simulink model "pipeline_sar_adc_v2"  (R2026a)
settings: Solver=FixedStepDiscrete  FixedStep=1e-9
values from neighbouring files (symbols this model uses):
  bit_1st = 6    [script_MonteCarlo.m]    (also in script_MonteCarlo_v2.m; script_spectrum.m; script_spectrum_v2.m)
  bit_2nd = 9    [script_MonteCarlo.m]    (also in script_MonteCarlo_v2.m; script_spectrum.m; script_spectrum_v2.m)
  CDAC_skew = 10e-9    (= 1e-08)    [script_MonteCarlo_v2.m]    (also in script_spectrum_v2.m = 1e-09)
  CMPno_1st = 0    [script_MonteCarlo.m]    (also in script_MonteCarlo_v2.m; script_spectrum.m; script_spectrum_v2.m)
  CMPno_2nd = 0    [script_MonteCarlo.m]    (also in script_MonteCarlo_v2.m; script_spectrum.m; script_spectrum_v2.m)
  CMPoff_1st = 0    [script_MonteCarlo.m]    (also in script_MonteCarlo_v2.m; script_spectrum.m; script_spectrum_v2.m)
  CMPoff_2nd = 0    [script_MonteCarlo.m]    (also in script_MonteCarlo_v2.m; script_spectrum.m; script_spectrum_v2.m)
  DAC_1st = DAC_1st_scaled(1 : (bit_1st + 1)) / (2^bit_1st)    [script_MonteCarlo.m]    (also in script_MonteCarlo_v2.m = DAC_1st_scaled(1 : bit_1st) / (2^(bit_1st-1)); script_spectrum.m; script_spectrum_v2.m = DAC_1st_scaled(1 : bit_1st) / (2^(bit_1st-1)))
  DAC_1st_v2 = DAC_big_scaled(1 : (bit_1st + 1)) / (2^bit_1st)    [script_MonteCarlo_v2.m]    (also in script_spectrum_v2.m)
  DAC_2nd = 0    [script_MonteCarlo.m]    (also in script_MonteCarlo_v2.m; script_spectrum.m; script_spectrum_v2.m)
  fin = (M / N) * fs    (= 488281.25)    [script_MonteCarlo.m]    (also in script_MonteCarlo_v2.m; script_spectrum.m; script_spectrum_v2.m = 292968.75)
  fs = 100e6    (= 100000000)    [script_MonteCarlo.m]    (also in script_MonteCarlo_v2.m; script_spectrum.m; script_spectrum_v2.m)
  mean_kTC = 0    [script_MonteCarlo.m]    (also in script_MonteCarlo_v2.m; script_spectrum.m; script_spectrum_v2.m)
  seed_kTC_1st = randi(1e6)    [script_MonteCarlo.m]    (also in script_MonteCarlo_v2.m; script_spectrum.m; script_spectrum_v2.m = randi(2^31))
  seed_kTC_2nd = randi(1e6)    [script_MonteCarlo.m]    (also in script_MonteCarlo_v2.m; script_spectrum.m; script_spectrum_v2.m = randi(2^31))
  seed_kTC_big = randi(1e6)    [script_MonteCarlo_v2.m]    (also in script_spectrum_v2.m = randi(2^31))
  var_kTC_1st = kTC_en_1st * sigma_kTC_1st^2    [script_MonteCarlo.m]    (also in script_MonteCarlo_v2.m; script_spectrum.m; script_spectrum_v2.m)
  var_kTC_2nd = kTC_en_2nd * sigma_kTC_2nd^2    [script_MonteCarlo.m]    (also in script_MonteCarlo_v2.m; script_spectrum.m; script_spectrum_v2.m)
  var_kTC_big = kTC_en_big * sigma_kTC_big^2    [script_MonteCarlo_v2.m]    (also in script_spectrum_v2.m)
  Vin = 0.95    [script_MonteCarlo.m]    (also in script_MonteCarlo_v2.m; script_parametric_analysis.m = Vin_array(idx); script_spectrum.m; script_spectrum_v2.m)
settings Model: Creator=오지훈  LastModifiedBy=오지훈

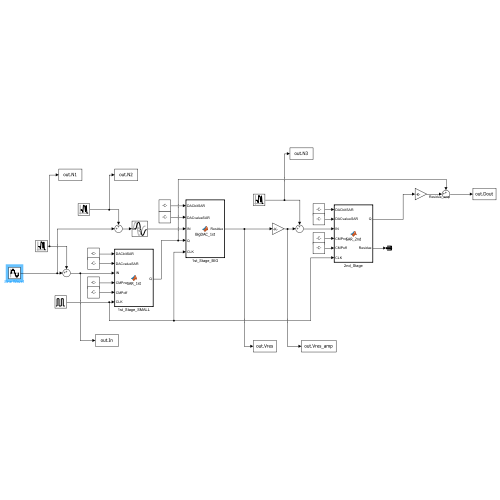
[thumbnail: Simulink's stored preview of the top-level diagram]
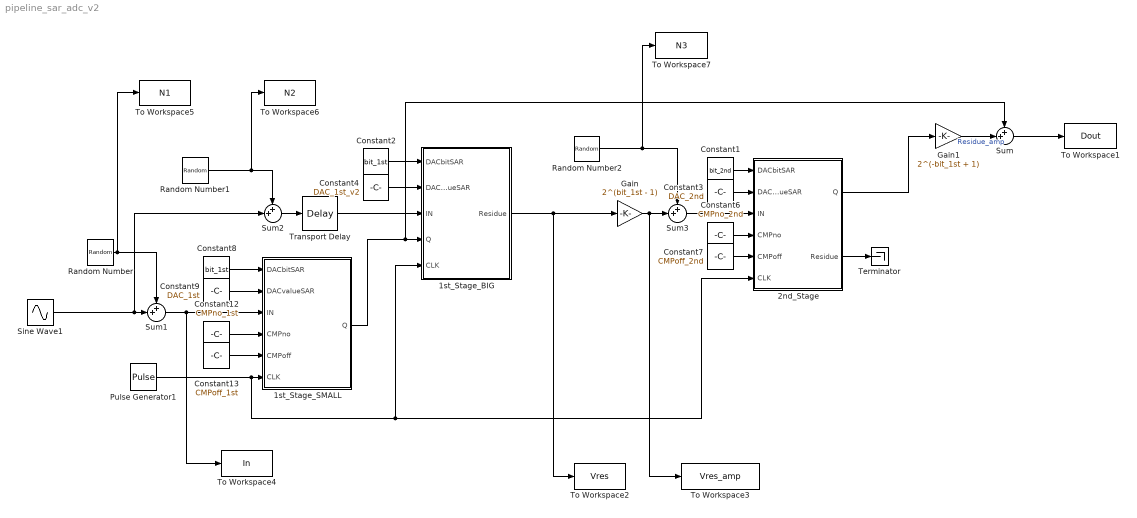
== system pipeline_sar_adc_v2 ==
  1st_Stage_BIG : MATLAB Function  TreatAsAtomicUnit=on
  1st_Stage_SMALL : MATLAB Function  TreatAsAtomicUnit=on
  2nd_Stage : MATLAB Function  TreatAsAtomicUnit=on
  Constant1 : Constant  Value=bit_2nd
  Constant12 : Constant  Value=CMPno_1st
  Constant13 : Constant  Value=CMPoff_1st
  Constant2 : Constant  Value=bit_1st
  Constant3 : Constant  Value=DAC_2nd
  Constant4 : Constant  Value=DAC_1st_v2
  Constant6 : Constant  Value=CMPno_2nd
  Constant7 : Constant  Value=CMPoff_2nd
  Constant8 : Constant  Value=bit_1st
  Constant9 : Constant  Value=DAC_1st
  Gain : Gain  Gain=2^(bit_1st - 1)
  Gain1 : Gain  Gain=2^(-bit_1st + 1)
  Pulse Generator1 : DiscretePulseGenerator  PulseType=Time based  Period=1/fs  PulseWidth=50
  Random Number : RandomNumber  Mean=mean_kTC  Variance=var_kTC_1st  Seed=seed_kTC_1st  SampleTime=1/fs
  Random Number1 : RandomNumber  Mean=mean_kTC  Variance=var_kTC_big  Seed=seed_kTC_big  SampleTime=1/fs
  Random Number2 : RandomNumber  Mean=mean_kTC  Variance=var_kTC_2nd  Seed=seed_kTC_2nd  SampleTime=1/fs
  Sine Wave1 : Sin  Amplitude=Vin  Frequency=2*pi*fin  SampleTime=CDAC_skew
  Sum{,1..3} (4 alike) : Sum  Inputs=++|
  Terminator : Terminator
  To Workspace1 : ToWorkspace  VariableName=Dout  SaveFormat=Timeseries  SampleTime=1/fs
  To Workspace2 : ToWorkspace  VariableName=Vres  SaveFormat=Timeseries  SampleTime=1/fs
  To Workspace3 : ToWorkspace  VariableName=Vres_amp  SaveFormat=Timeseries  SampleTime=1/fs
  To Workspace4 : ToWorkspace  VariableName=In  SaveFormat=Timeseries  SampleTime=1/fs
  To Workspace5 : ToWorkspace  VariableName=N1  SaveFormat=Timeseries  SampleTime=1/fs
  To Workspace6 : ToWorkspace  VariableName=N2  SaveFormat=Timeseries  SampleTime=1/fs
  To Workspace7 : ToWorkspace  VariableName=N3  SaveFormat=Timeseries  SampleTime=1/fs
  Transport Delay : TransportDelay  DelayTime=CDAC_skew
  wires:
  Sum1/1 -> To Workspace4/1, 1st_Stage_SMALL/3(IN)
  2nd_Stage/2(Residue) -> Terminator/1
  Constant3/1 -> 2nd_Stage/2(DACvalueSAR)
  Constant4/1 -> 1st_Stage_BIG/2(DACvalueSAR)
  Constant2/1 -> 1st_Stage_BIG/1(DACbitSAR)
  1st_Stage_BIG/1(Residue) -> Gain/1, To Workspace2/1
  Constant1/1 -> 2nd_Stage/1(DACbitSAR)
  Constant7/1 -> 2nd_Stage/5(CMPoff)
  Constant13/1 -> 1st_Stage_SMALL/5(CMPoff)
  Constant6/1 -> 2nd_Stage/4(CMPno)
  Sum/1 -> To Workspace1/1
  Constant12/1 -> 1st_Stage_SMALL/4(CMPno)
  Constant9/1 -> 1st_Stage_SMALL/2(DACvalueSAR)
  Gain/1 -> To Workspace3/1, Sum3/2
  Gain1/1 -> Sum/2  "Residue_amp"
  Constant8/1 -> 1st_Stage_SMALL/1(DACbitSAR)
  2nd_Stage/1(Q) -> Gain1/1
  Pulse Generator1/1 -> 2nd_Stage/6(CLK), 1st_Stage_BIG/5(CLK), 1st_Stage_SMALL/6(CLK)
  1st_Stage_SMALL/1(Q) -> 1st_Stage_BIG/4(Q), Sum/1
  Sine Wave1/1 -> Sum2/2, Sum1/2
  Random Number/1 -> To Workspace5/1, Sum1/1
  Sum2/1 -> Transport Delay/1
  Random Number1/1 -> To Workspace6/1, Sum2/1
  Sum3/1 -> 2nd_Stage/3(IN)
  Random Number2/1 -> To Workspace7/1, Sum3/1
  Transport Delay/1 -> 1st_Stage_BIG/3(IN)

== matlab function pipeline_sar_adc_v2/1st_Stage_SMALL ==
  data: DACbitSAR input; Q output; DACvalueSAR input; IN input; CMPno input; CMPoff input; CLK input
function Q = SAR_1st(DACbitSAR, DACvalueSAR, IN, CMPno, CMPoff, CLK)
persistent last_CLK Q_hold
if isempty(last_CLK)
    last_CLK = 0;
    Q_hold = 0;
end
if (last_CLK == 0) && (CLK == 1)
    current_residue = IN;
    Q_partial_sum = 0;
    len_DAC = length(DACvalueSAR);
    
    % --- SAR 5번 판정 (residue 5번 갱신) ---
    for i = 1:DACbitSAR-1
        CMP_threshold = CMPno * randn(1) + CMPoff;
        current_idx = len_DAC - i + 1;
        current_dac = DACvalueSAR(current_idx);
        bit_weight = 2^(-(i-1));
        if current_residue >= CMP_threshold
            current_residue = current_residue - current_dac;
            Q_partial_sum = Q_partial_sum + 1 * bit_weight;
        else
            current_residue = current_residue + current_dac;
        end
    end
    
    % --- Residue 확정 후 마지막 판정 (Q에만 반영, residue 갱신 없음) ---
    CMP_threshold = CMPno * randn(1) + CMPoff;
    bit_weight = 2^(-(DACbitSAR-1));   % 마지막 bit weight = 2^-5
    if current_residue >= CMP_threshold
        Q_partial_sum = Q_partial_sum + 1 * bit_weight;
    end
    
    Q_hold = Q_partial_sum - 1;
end
Q = Q_hold;
last_CLK = CLK;
end

== matlab function pipeline_sar_adc_v2/1st_Stage_BIG ==
  data: DACbitSAR input; DACvalueSAR input; IN input; Q input; Residue output; CLK input
function Residue = BigDAC_1st(DACbitSAR, DACvalueSAR, IN, Q, CLK)
% Big DAC (1st stage) — 판정 없음. Small DAC의 코드(Q)를 받아 residue만 생성.
% 에러: 커패시터 미스매치(DACvalueSAR에 반영).
% 비교기 offset/noise 없음 (이 블록에는 비교기가 없음).
persistent last_CLK Residue_hold
if isempty(last_CLK)
    last_CLK = 0;
    Residue_hold = 0;
end

if (last_CLK == 0) && (CLK == 1)
    current_residue = IN;
    len_DAC = length(DACvalueSAR);

    % ---- Q로부터 Small DAC의 비트 결정을 복원 (재비교 안 함) ----
    Q_partial_sum = Q + 1;              % small의 -1 스케일링 역산
    remaining = Q_partial_sum;

    for i = 1:DACbitSAR
        bit_weight = 2^(-(i-1));
        current_idx = len_DAC - i + 1;
        current_dac = DACvalueSAR(current_idx);   % 미스매치 포함 실제 값

        % small이 이 비트를 1로 정했는지 복원
        if remaining >= bit_weight
            bit = 1;
            remaining = remaining - bit_weight;
        else
            bit = 0;
        end

        % small의 결정 그대로 따라 residue 갱신
        if bit == 1
            current_residue = current_residue - current_dac;
        else
            current_residue = current_residue + current_dac;
        end
    end

    Residue_hold = current_residue;
end

Residue = Residue_hold;
last_CLK = CLK;
end

== matlab function pipeline_sar_adc_v2/2nd_Stage ==
  data: DACbitSAR input; Q output; DACvalueSAR input; IN input; CMPno input; CMPoff input; Residue output; CLK input
function [Q, Residue] = SAR_2nd(DACbitSAR, DACvalueSAR, IN, CMPno, CMPoff, CLK)
persistent last_CLK Q_hold Residue_hold

if isempty(last_CLK)
    last_CLK = 0;
    Q_hold = 0;
    Residue_hold = 0;
end

if (last_CLK == 0) && (CLK == 1)
    
    current_residue = IN; 
    Q_partial_sum = 0;    % ★ Partial sum을 누적할 변수 초기화
    len_DAC = length(DACvalueSAR); 
    
    for i = 1:DACbitSAR
        CMP_threshold = CMPno * randn(1) + CMPoff;
        
        current_idx = len_DAC - i + 1; 
        current_dac = DACvalueSAR(current_idx);
        
        % 각 비트 자리에 해당하는 이진 가중치 (1, 0.5, 0.25, 0.125 ...)
        bit_weight = 2^(-(i-1)); 
        
        if current_residue >= CMP_threshold
            current_residue = current_residue - current_dac;
            % ★ 비트가 1일 때, 가중치(bit_weight)를 partial sum에 바로 누적
            Q_partial_sum = Q_partial_sum + 1 * bit_weight;
        else
            current_residue = current_residue + current_dac;
            % 비트가 0일 때는 0 * bit_weight 이므로 누적 생략 (혹은 +0)
        end
    end
    
    % ★ 최종 스케일링: [2 곱하기]를 빼고 [1만 빼는] 규칙 적용
    % Virtuoso 수식의 ((VT(MSB) + VT(MSB-1)/2 + ...) - 1) 과 완벽히 매칭됩니다.
    Q_hold = Q_partial_sum - 1;
    
    Residue_hold = current_residue;
end

Q = Q_hold;
Residue = Residue_hold;
last_CLK = CLK;
end
